simulink model "rtwdemo_rsim_vdp"  (Simulink 7.6)
settings: Solver=ode45  StartTime=0.0  StopTime=50.0  RelTol=1e-6  SampleTimeConstraint=STIndependent
PreLoadFcn:
  | INIT_X1 = 2;
  | INIT_X2 = 0;
  | MU  = 1;
CloseFcn:
  | clear INIT_X1 INIT_X2  MU;
settings Model: Creator=The MathWorks Inc.  ExtModeAutoUpdateStatusClock=off
settings OptimizationCC: InlineParams=on  InlineInvariantSignals=on  EfficientFloat2IntCast=on  EfficientMapNaN2IntZero=off
settings DebuggingCC: SolverPrmCheckMsg=none  StrictBusMsg=ErrorOnBusTreatedAsVector
settings HardwareCC: ProdIntDivRoundTo=Zero  ProdEndianess=LittleEndian  ProdHWDeviceType=Generic->32-bit Embedded Processor  TargetHWDeviceType=Generic->32-bit Embedded Processor
settings RTWCC: SystemTargetFile=rsim.tlc  TLCOptions=-p0  TemplateMakefile=rsim_default_tmf  Description=Rapid Simulation Target  RTWVerbose=off  ProcessScript=rsim_make_rtw_hook
settings RSimTargetCC: TargetFcnLib=ansi_tfl_tmw.mat  TargetFunctionLibrary=ANSI_C  ERTMultiwordTypeDef=System defined  ERTCodeCoverageTool=None  ERTMultiwordLength=256  IsPILTarget=off  EnableShiftOperators=on  PortableWordSizes=off

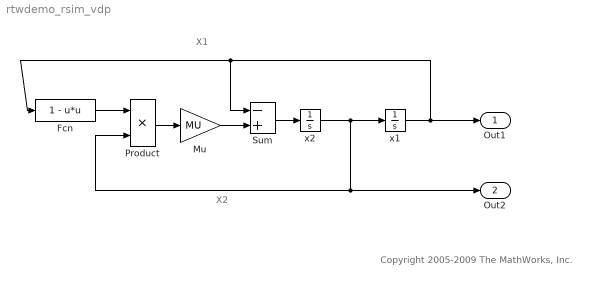
== system rtwdemo_rsim_vdp ==
  note: X2
  note: X1
  note: Copyright 2005-2009 The MathWorks, Inc.
  Fcn : Fcn  Expr=1 - u*u
  Mu : Gain  Gain=MU  SaturateOnIntegerOverflow=on  OutDataTypeStr=Inherit: Same as input  ParamDataTypeStr=Inherit: Same as input
  Product : Product  SaturateOnIntegerOverflow=on  RndMeth=Zero  InputSameDT=on  OutDataTypeStr=Inherit: Same as first input
  Sum : Sum  Inputs=-+  SaturateOnIntegerOverflow=on  InputSameDT=on  OutDataTypeStr=Inherit: Same as first input
  x1 : Integrator  InitialCondition=INIT_X1
  x2 : Integrator  InitialCondition=INIT_X2
  Out1 : Outport  InitialOutput=0
  Out2 : Outport  Port=2  InitialOutput=0
  wires:
  Product/1 -> Mu/1
  Mu/1 -> Sum/2
  Sum/1 -> x2/1
  x2/1 -> x1/1, Out2/1, Product/2
  x1/1 -> Out1/1, Fcn/1, Sum/1
  Fcn/1 -> Product/1
